simulink model "sine_cos_gen"  (R2019b)
settings: Solver=VariableStepAuto  StartTime=0.0  StopTime=10  RelTol=1e-3
libraries: simulink x1
settings Model: Creator=Tris  LastModifiedBy=Tris

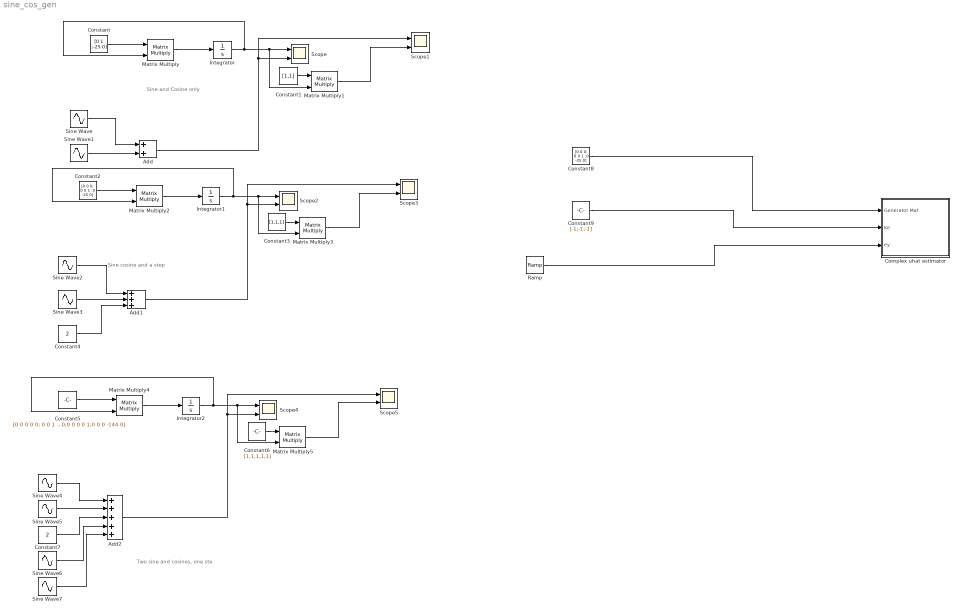
== system sine_cos_gen ==
  note: Two sine and cosines, one ste
  note: Sine cosine and a step
  note: Sine and Cosine only
  Add : Sum
  Add1 : Sum  Inputs=+++
  Add2 : Sum  Inputs=+++++
  Complex uhat estimator : Subsystem
  Constant : Constant  Value=[0 1 ;-25 0]
  Constant1 : Constant  Value=[1,1]  VectorParams1D=off
  Constant2 : Constant  Value=[0 0 0; 0 0 1 ;0 -25 0]
  Constant3 : Constant  Value=[1,1,1]  VectorParams1D=off
  Constant4 : Constant  Value=2
  Constant5 : Constant  Value=[0 0 0 0 0; 0 0 1 0 0;0 -25 0 0 0;0 0 0 0 1;0 0 0 -144 0]
  Constant6 : Constant  Value=[1,1,1,1,1]  VectorParams1D=off
  Constant7 : Constant  Value=2
  Constant8 : Constant  Value=[0 0 0; 0 0 1 ;0 -25 0]
  Constant9 : Constant  Value=[-1;-1;-1]
  Integrator : Integrator  InitialCondition=[0;1]
  Integrator1 : Integrator  InitialCondition=[2;0;1]
  Integrator2 : Integrator  InitialCondition=[2;0;1;0;1]
  Matrix Multiply{,1..5} (6 alike) : Product  Multiplication=Matrix(*)
  Ramp : simulink/Sources/Ramp  slope=0  start=0  InitialOutput=0  VectorParams1D=off
  Scope{,1..5} (6 alike) : Scope  NumInputPorts=2
  Sine Wave : Sin  Amplitude=1/5  Frequency=5  SampleTime=0
  Sine Wave1 : Sin  Frequency=5  Phase=pi/2  SampleTime=0
  Sine Wave2 : Sin  Amplitude=1/5  Frequency=5  SampleTime=0
  Sine Wave3 : Sin  Frequency=5  Phase=pi/2  SampleTime=0
  Sine Wave4 : Sin  Amplitude=1/5  Frequency=5  SampleTime=0
  Sine Wave5 : Sin  Frequency=5  Phase=pi/2  SampleTime=0
  Sine Wave6 : Sin  Amplitude=1/12  Frequency=12  SampleTime=0
  Sine Wave7 : Sin  Frequency=12  Phase=pi/2  SampleTime=0
  wires:
  Constant/1 -> Matrix Multiply/1
  Matrix Multiply/1 -> Integrator/1
  Integrator/1 -> Matrix Multiply1/2, Scope/1, Matrix Multiply/2
  Add/1 -> Scope1/1, Scope/2
  Constant1/1 -> Matrix Multiply1/1
  Matrix Multiply1/1 -> Scope1/2
  Sine Wave/1 -> Add/1
  Sine Wave1/1 -> Add/2
  Sine Wave3/1 -> Add1/2
  Matrix Multiply2/1 -> Integrator1/1
  Constant2/1 -> Matrix Multiply2/1
  Integrator1/1 -> Matrix Multiply3/2, Scope2/1, Matrix Multiply2/2
  Add1/1 -> Scope3/1, Scope2/2
  Sine Wave2/1 -> Add1/1
  Matrix Multiply3/1 -> Scope3/2
  Constant3/1 -> Matrix Multiply3/1
  Constant4/1 -> Add1/3
  Matrix Multiply5/1 -> Scope5/2
  Sine Wave4/1 -> Add2/1
  Constant6/1 -> Matrix Multiply5/1
  Add2/1 -> Scope5/1, Scope4/2
  Integrator2/1 -> Matrix Multiply5/2, Scope4/1, Matrix Multiply4/2
  Constant7/1 -> Add2/3
  Constant5/1 -> Matrix Multiply4/1
  Sine Wave5/1 -> Add2/2
  Matrix Multiply4/1 -> Integrator2/1
  Sine Wave6/1 -> Add2/4
  Sine Wave7/1 -> Add2/5
  Constant8/1 -> Complex uhat estimator/1(Generator Mat)
  Constant9/1 -> Complex uhat estimator/2(Ke)
  Ramp/1 -> Complex uhat estimator/3(ey)

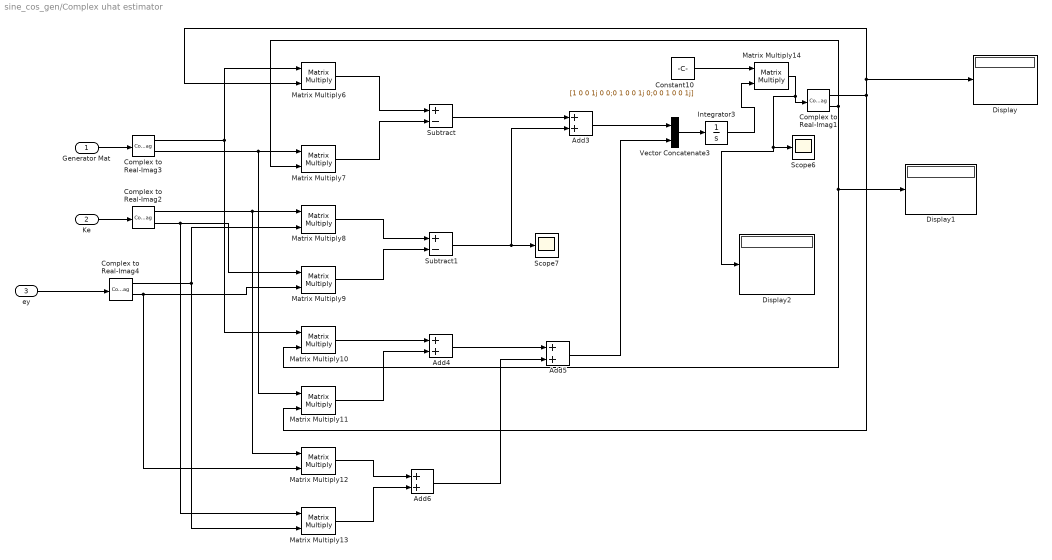
== system sine_cos_gen/Complex uhat estimator ==
  Generator Mat : Inport
  Ke : Inport  Port=2
  ey : Inport  Port=3
  Add{3..6} (4 alike) : Sum
  Complex to Real-Imag{1..4} (4 alike) : ComplexToRealImag
  Constant10 : Constant  Value=[1 0 0 1j 0 0;0 1 0 0 1j 0;0 0 1 0 0 1j]  VectorParams1D=off
  Display : Display
  Display1 : Display
  Display2 : Display
  Integrator3 : Integrator  InitialCondition=[2;0;1;0;0;0]
  Matrix Multiply{6..14} (9 alike) : Product  Multiplication=Matrix(*)
  Scope6 : Scope
  Scope7 : Scope
  Subtract : Sum  Inputs=+-
  Subtract1 : Sum  Inputs=+-
  Vector Concatenate3 : Concatenate  Mode=Multidimensional array
  wires:
  Matrix Multiply8/1 -> Subtract1/1
  Complex to Real-Imag1/1 -> Matrix Multiply6/2, Display/1, Matrix Multiply11/2
  Ke/1 -> Complex to Real-Imag2/1
  Complex to Real-Imag3/1 -> Matrix Multiply6/1, Matrix Multiply10/1
  Matrix Multiply11/1 -> Add4/2
  Matrix Multiply12/1 -> Add6/1
  Subtract1/1 -> Scope7/1, Add3/2
  Complex to Real-Imag2/1 -> Matrix Multiply12/1, Matrix Multiply8/1
  Matrix Multiply10/1 -> Add4/1
  Complex to Real-Imag4/2 -> Matrix Multiply12/2, Matrix Multiply9/2
  Add4/1 -> Add5/1
  Add6/1 -> Add5/2
  Complex to Real-Imag1/2 -> Display1/1, Matrix Multiply10/2, Matrix Multiply7/2
  Complex to Real-Imag2/2 -> Matrix Multiply13/1, Matrix Multiply9/1
  Generator Mat/1 -> Complex to Real-Imag3/1
  Complex to Real-Imag4/1 -> Matrix Multiply8/2, Matrix Multiply13/2
  Complex to Real-Imag3/2 -> Matrix Multiply11/1, Matrix Multiply7/1
  Vector Concatenate3/1 -> Integrator3/1
  Add3/1 -> Vector Concatenate3/1
  Constant10/1 -> Matrix Multiply14/1
  Matrix Multiply13/1 -> Add6/2
  Subtract/1 -> Add3/1
  Matrix Multiply7/1 -> Subtract/2
  Matrix Multiply14/1 -> Display2/1, Scope6/1, Complex to Real-Imag1/1
  Add5/1 -> Vector Concatenate3/2
  Matrix Multiply6/1 -> Subtract/1
  Integrator3/1 -> Matrix Multiply14/2
  Matrix Multiply9/1 -> Subtract1/2
  ey/1 -> Complex to Real-Imag4/1
